simulink model "view"  (Simulink 6.1)
settings: Solver=ode3  StartTime=0.0  StopTime=10.0  FixedStep=0.01  RelTol=1e-3
settings Model: LastModifiedBy=okawa
settings DebuggingCC: SolverPrmCheckMsg=warning

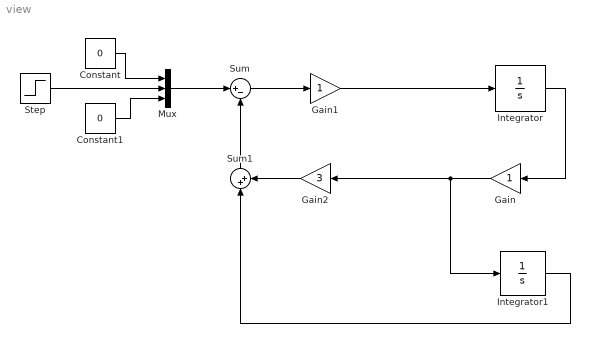
== system view ==
  Constant : Constant  Value=0
  Constant1 : Constant  Value=0
  Gain : Gain  Orientation=left
  Gain1 : Gain
  Gain2 : Gain  Orientation=left  Gain=3
  Integrator : Integrator
  Integrator1 : Integrator
  Mux : Mux  Inputs=3
  Step : Step  SampleTime=0
  Sum : Sum  Inputs=|+-
  Sum1 : Sum  Orientation=up  Inputs=|++
  wires:
  Constant/1 -> Mux/1
  Step/1 -> Mux/2
  Constant1/1 -> Mux/3
  Integrator/1 -> Gain/1
  Gain/1 -> Integrator1/1, Gain2/1
  Gain1/1 -> Integrator/1
  Sum/1 -> Gain1/1
  Mux/1 -> Sum/1
  Sum1/1 -> Sum/2
  Integrator1/1 -> Sum1/1
  Gain2/1 -> Sum1/2
